simulink subsystem "Final_Project_PreBusUnpack_20260601_105527"  (R2024a)
settings: Solver=VariableStepAuto  StartTime=0.0  StopTime=10.0  RelTol=1e-3
values from neighbouring files (symbols this model uses):
  D = hypot(Ep(:,1)-Tp(:,1)',Ep(:,2)-Tp(:,2)')    [pp_compare_stage.m]    (also in pp_diag_path.m; pp_t09_clear.m = hypot(Ep(:,1)-Tperim(:,1)', Ep(:,2)-Tperim(:,2)'); pp_tune2.m)
undefined symbols (not defined in the file or in its folder): waypoints
libraries: CarMaker4SL x116, simulink x1
(part 4 of 7)

== matlab function Final_Project_PreBusUnpack_20260601_105527/Driving_Module_Ver.3_PSH/Subsystem/Ego_Detector ==
  data: ego_state input; ego_lane_id output; lanes input; target_lane_fb input; ego_cross_track_err output; ego_head_err output; ego_max_curvature output; park_cmd input
function [ego_lane_id, ego_cross_track_err, ego_head_err, ego_max_curvature] = Ego_Detector(ego_state, lanes, target_lane_fb, park_cmd)
%#codegen

    % ============================================================
    % 1. EgoStateBus unpack
    % ============================================================
    ego_x   = ego_state.Car_Fr1_tx;
    ego_y   = ego_state.Car_Fr1_ty;
    ego_yaw = ego_state.Car_Fr1_rz;

    % ============================================================
    % 2. ParsedLaneBus unpack - 5차선
    % ============================================================
    x1 = lanes.x1;  y1 = lanes.y1;
    x2 = lanes.x2;  y2 = lanes.y2;
    x3 = lanes.x3;  y3 = lanes.y3;
    x4 = lanes.x4;  y4 = lanes.y4;
    x5 = lanes.x5;  y5 = lanes.y5;

    % lane5 좌측 보정
    L5_OFFSET = 1.0;
    x5 = x5 + L5_OFFSET;

    % ============================================================
    % 3. 현재 ego가 가장 가까운 차선 판단
    % ============================================================
    d1 = nearest_d2(x1, y1, ego_x, ego_y);
    d2 = nearest_d2(x2, y2, ego_x, ego_y);
    d3 = nearest_d2(x3, y3, ego_x, ego_y);
    d4 = nearest_d2(x4, y4, ego_x, ego_y);
    d5 = nearest_d2(x5, y5, ego_x, ego_y);

    ego_lane_id = int32(1);
    dmin = d1;

    if d2 < dmin
        dmin = d2;
        ego_lane_id = int32(2);
    end

    if d3 < dmin
        dmin = d3;
        ego_lane_id = int32(3);
    end

    if d4 < dmin
        dmin = d4;
        ego_lane_id = int32(4);
    end

    if d5 < dmin
        ego_lane_id = int32(5);
    end

    % ============================================================
    % 4. target_lane 보호
    % ============================================================
    target_lane = int32(target_lane_fb);

    if target_lane < int32(1)
        target_lane = int32(1);
    elseif target_lane > int32(5)
        target_lane = int32(5);
    end

    % ============================================================
    % 5. 주차 진입 구간에서는 preview step 축소
    % ============================================================
    if park_cmd == int32(1) && ...
       (target_lane == int32(4) || target_lane == int32(5))
        LOOK_STEP = int32(2);
    else
        LOOK_STEP = int32(5);
    end

    % ============================================================
    % 6. target lane 기준 오차 / 곡률 계산
    % ============================================================
    if target_lane == int32(1)

        [ego_cross_track_err, ego_head_err, ego_max_curvature] = process_lane_closed( ...
            x1, y1, ego_x, ego_y, ego_yaw, LOOK_STEP);

    elseif target_lane == int32(2)

        [ego_cross_track_err, ego_head_err, ego_max_curvature] = process_lane_closed( ...
            x2, y2, ego_x, ego_y, ego_yaw, LOOK_STEP);

    elseif target_lane == int32(3)

        [ego_cross_track_err, ego_head_err, ego_max_curvature] = process_lane_closed( ...
            x3, y3, ego_x, ego_y, ego_yaw, LOOK_STEP);

    elseif target_lane == int32(4)

        [ego_cross_track_err, ego_head_err, ego_max_curvature] = process_lane_open( ...
            x4, y4, ego_x, ego_y, ego_yaw, LOOK_STEP);

    else

        [ego_cross_track_err, ego_head_err, ego_max_curvature] = process_lane_open( ...
            x5, y5, ego_x, ego_y, ego_yaw, LOOK_STEP);

    end

end


function d2 = nearest_d2(xa, ya, ex, ey)
%#codegen

    d2 = 1e12;
    N  = int32(numel(xa));

    for i = 1:N
        dxk = xa(i) - ex;
        dyk = ya(i) - ey;
        v   = dxk*dxk + dyk*dyk;

        if v < d2
            d2 = v;
        end
    end

end


function [ego_cross_track_err, ego_head_err, ego_max_curvature] = process_lane_open(xa, ya, ex, ey, eyaw, LOOK_STEP)
%#codegen

    N = int32(numel(xa));

    best_i  = int32(1);
    best_d2 = 1e12;

    for i = 1:N
        dxk = xa(i) - ex;
        dyk = ya(i) - ey;
        v   = dxk*dxk + dyk*dyk;

        if v < best_d2
            best_d2 = v;
            best_i  = i;
        end
    end

    look_i = best_i + LOOK_STEP;

    if look_i > N
        look_i = N;
    end

    if look_i > best_i

        path_yaw = atan2( ...
            ya(look_i) - ya(best_i), ...
            xa(look_i) - xa(best_i));

    elseif best_i > int32(1)

        path_yaw = atan2( ...
            ya(best_i) - ya(best_i - int32(1)), ...
            xa(best_i) - xa(best_i - int32(1)));

    else

        path_yaw = eyaw;

    end

    dxr = ex - xa(best_i);
    dyr = ey - ya(best_i);

    ego_cross_track_err = -sin(path_yaw) * dxr + cos(path_yaw) * dyr;

    ego_head_err = wrap_pi(path_yaw - eyaw);

    ego_max_curvature = 0.0;
    STEP = int32(5);

    for kk = 0:4
        base_i = best_i + int32(kk) * STEP;

        i1 = base_i;
        i2 = base_i + STEP;
        i3 = base_i + int32(2) * STEP;

        if i1 > N
            i1 = N;
        end

        if i2 > N
            i2 = N;
        end

        if i3 > N
            i3 = N;
        end

        if i1 < i2 && i2 < i3

            yaw1 = atan2( ...
                ya(i2) - ya(i1), ...
                xa(i2) - xa(i1));

            yaw2 = atan2( ...
                ya(i3) - ya(i2), ...
                xa(i3) - xa(i2));

            dyaw = wrap_pi(yaw2 - yaw1);

            ds = sqrt( ...
                (xa(i3) - xa(i1))^2 + ...
                (ya(i3) - ya(i1))^2);

            if ds > 0.1
                kappa = abs(dyaw) / ds;

                if kappa > ego_max_curvature
                    ego_max_curvature = kappa;
                end
            end
        end
    end

end


function [ego_cross_track_err, ego_head_err, ego_max_curvature] = process_lane_closed(xa, ya, ex, ey, eyaw, LOOK_STEP)
%#codegen

    N = int32(numel(xa));

    best_i  = int32(1);
    best_d2 = 1e12;

    for i = 1:N
        dxk = xa(i) - ex;
        dyk = ya(i) - ey;
        v   = dxk*dxk + dyk*dyk;

        if v < best_d2
            best_d2 = v;
            best_i  = i;
        end
    end

    look_i = wrap_idx(best_i + LOOK_STEP, N);

    path_yaw = atan2( ...
        ya(look_i) - ya(best_i), ...
        xa(look_i) - xa(best_i));

    dxr = ex - xa(best_i);
    dyr = ey - ya(best_i);

    ego_cross_track_err = -sin(path_yaw) * dxr + cos(path_yaw) * dyr;

    ego_head_err = wrap_pi(path_yaw - eyaw);

    ego_max_curvature = 0.0;
    STEP = int32(5);

    for kk = 0:4
        base_i = wrap_idx(best_i + int32(kk) * STEP, N);

        i1 = base_i;
        i2 = wrap_idx(base_i + STEP, N);
        i3 = wrap_idx(base_i + int32(2) * STEP, N);

        yaw1 = atan2( ...
            ya(i2) - ya(i1), ...
            xa(i2) - xa(i1));

        yaw2 = atan2( ...
            ya(i3) - ya(i2), ...
            xa(i3) - xa(i2));

        dyaw = wrap_pi(yaw2 - yaw1);

        ds = sqrt( ...
            (xa(i3) - xa(i1))^2 + ...
            (ya(i3) - ya(i1))^2);

        if ds > 0.1
            kappa = abs(dyaw) / ds;

            if kappa > ego_max_curvature
                ego_max_curvature = kappa;
            end
        end
    end

end


function idx = wrap_idx(idx_in, N)
%#codegen
    idx = idx_in;

    while idx > N
        idx = idx - N;
    end

    while idx < int32(1)
        idx = idx + N;
    end

end


function a = wrap_pi(a)
%#codegen

    while a > pi
        a = a - 2.0*pi;
    end

    while a < -pi
        a = a + 2.0*pi;
    end

end

== stateflow chart Final_Project_PreBusUnpack_20260601_105527/Chart ==
  (default) -> (junction 1)
  (junction 1) -> (junction 3) [order 1] : [mod(i,10) == 0]
      | {do_Logic_10ms;}
  (junction 1) -> (junction 7) [order 2]
  (junction 3) -> (junction 5)
  (junction 5) -> (junction 7)
  (junction 7) -> (junction 10)
  (junction 10) -> (junction 12) [order 1] : [mod(i, 50) == 0]
      | {do_Logic_50ms;}
  (junction 10) -> (junction 18) [order 2]
  (junction 12) -> (junction 16)
  (junction 16) -> (junction 18)
  (junction 18) -> (junction 25)
  (junction 25) -> (junction 27) [order 1] : [mod(i,100) == 0]
      | {do_Logic_100ms;}
  (junction 25) -> (junction 21) [order 2]
  (junction 27) -> (junction 29) : {i = 0;}
  (junction 29) -> (junction 21)
  (junction 21) -> (junction 32) : {i = i +1;}
  data: i local =0
  events: do_Logic_10ms output FUNCTION_CALL_EVENT; do_Logic_50ms output FUNCTION_CALL_EVENT; do_Logic_100ms output FUNCTION_CALL_EVENT

== matlab function Final_Project_PreBusUnpack_20260601_105527/Driving_Module_Ver.3_PSH/Subsystem/Traffic_Detector ==
  data: ego_state input Bus: EgoStateBus; lead_dist output double; lanes input Bus: ParsedLaneBus; traffic input; target_speed input double; ego_lane_id input int32; lead_speed output double; left_clear output boolean; right_clear output boolean
function [lead_dist, lead_speed, left_clear, right_clear] = Traffic_Detector(ego_state, lanes, traffic, target_speed, ego_lane_id)
%#codegen
% traffic : Obstacle_Info_Bus
% 내부 구조 예:
%   traffic.t16.x, traffic.t16.y, traffic.t16.vx, traffic.t16.vy
%   ...
%   traffic.t28.x, traffic.t28.y, traffic.t28.vx, traffic.t28.vy
%
% 주의:
%   target_speed는 배선 호환용으로 남겨두지만, 거리 판단에는 ego_v를 사용함.

    unused_target_speed = target_speed; %#ok<NASGU>

    % ============================================================
    % 0. 출력 초기화
    % ============================================================
    lead_dist   = 1e9;
    lead_speed  = 0.0;
    left_clear  = true;
    right_clear = true;
    ego_lane    = int32(ego_lane_id);

    % ============================================================
    % 1. Ego unpack
    % ============================================================
    ego_x = ego_state.Car_Fr1_tx;
    ego_y = ego_state.Car_Fr1_ty;
    ego_v = ego_state.Ego_V;

    % ============================================================
    % 2. Lane unpack - 5차선
    % ============================================================
    x1 = lanes.x1; y1 = lanes.y1;
    x2 = lanes.x2; y2 = lanes.y2;
    x3 = lanes.x3; y3 = lanes.y3;
    x4 = lanes.x4; y4 = lanes.y4;
    x5 = lanes.x5; y5 = lanes.y5;

    % detector와 lane5 기준을 맞추기 위한 보정
    L5_OFFSET = 1.0;
    x5 = x5 + L5_OFFSET;

    % ============================================================
    % 3. Ego 속도 기반 가변 탐색/안전거리
    % ============================================================
    v_ego_gap = abs(ego_v);

    if v_ego_gap > 60.0
        v_ego_gap = v_ego_gap / 3.6;
    end

    LOOK_FRONT = calcLookFront(v_ego_gap);

    CLEAR_BACK_MIN = 5.0;
    CLEAR_BACK_TG  = 0.5;
    CLEAR_BACK_MAX = 35.0;

    CLEAR_BACK = CLEAR_BACK_MIN + CLEAR_BACK_TG * v_ego_gap;

    if CLEAR_BACK > CLEAR_BACK_MAX
        CLEAR_BACK = CLEAR_BACK_MAX;
    end

    CLEAR_FRONT_MIN = 15.0;
    CLEAR_FRONT_TG  = 0.9;
    CLEAR_FRONT_MAX = 70.0;

    CLEAR_FRONT = CLEAR_FRONT_MIN + CLEAR_FRONT_TG * v_ego_gap;

    if CLEAR_FRONT > CLEAR_FRONT_MAX
        CLEAR_FRONT = CLEAR_FRONT_MAX;
    end

    % ============================================================
    % 4. Init
    % ============================================================
    lead_dist  = 1e9;
    lead_speed = v_ego_gap;

    left_clear  = true;
    right_clear = true;

    if ego_lane >= int32(5)
        left_clear = false;
    end

    if ego_lane <= int32(1)
        right_clear = false;
    end

    % ============================================================
    % 5. Traffic_Info_16_Bus ~ Traffic_Info_28_Bus 직접 처리
    % ============================================================
    [lead_dist, lead_speed, left_clear, right_clear] = check_one_signal( ...
        traffic.t16.x, traffic.t16.y, traffic.t16.vx, traffic.t16.vy, true, ...
        ego_x, ego_y, ego_lane, ...
        x1,y1,x2,y2,x3,y3,x4,y4,x5,y5, ...
        lead_dist, lead_speed, left_clear, right_clear, ...
        LOOK_FRONT, CLEAR_BACK, CLEAR_FRONT);

    [lead_dist, lead_speed, left_clear, right_clear] = check_one_signal( ...
        traffic.t17.x, traffic.t17.y, traffic.t17.vx, traffic.t17.vy, true, ...
        ego_x, ego_y, ego_lane, ...
        x1,y1,x2,y2,x3,y3,x4,y4,x5,y5, ...
        lead_dist, lead_speed, left_clear, right_clear, ...
        LOOK_FRONT, CLEAR_BACK, CLEAR_FRONT);

    [lead_dist, lead_speed, left_clear, right_clear] = check_one_signal( ...
        traffic.t18.x, traffic.t18.y, traffic.t18.vx, traffic.t18.vy, true, ...
        ego_x, ego_y, ego_lane, ...
        x1,y1,x2,y2,x3,y3,x4,y4,x5,y5, ...
        lead_dist, lead_speed, left_clear, right_clear, ...
        LOOK_FRONT, CLEAR_BACK, CLEAR_FRONT);

    [lead_dist, lead_speed, left_clear, right_clear] = check_one_signal( ...
        traffic.t19.x, traffic.t19.y, traffic.t19.vx, traffic.t19.vy, true, ...
        ego_x, ego_y, ego_lane, ...
        x1,y1,x2,y2,x3,y3,x4,y4,x5,y5, ...
        lead_dist, lead_speed, left_clear, right_clear, ...
        LOOK_FRONT, CLEAR_BACK, CLEAR_FRONT);

    [lead_dist, lead_speed, left_clear, right_clear] = check_one_signal( ...
        traffic.t20.x, traffic.t20.y, traffic.t20.vx, traffic.t20.vy, true, ...
        ego_x, ego_y, ego_lane, ...
        x1,y1,x2,y2,x3,y3,x4,y4,x5,y5, ...
        lead_dist, lead_speed, left_clear, right_clear, ...
        LOOK_FRONT, CLEAR_BACK, CLEAR_FRONT);

    [lead_dist, lead_speed, left_clear, right_clear] = check_one_signal( ...
        traffic.t21.x, traffic.t21.y, traffic.t21.vx, traffic.t21.vy, true, ...
        ego_x, ego_y, ego_lane, ...
        x1,y1,x2,y2,x3,y3,x4,y4,x5,y5, ...
        lead_dist, lead_speed, left_clear, right_clear, ...
        LOOK_FRONT, CLEAR_BACK, CLEAR_FRONT);

    [lead_dist, lead_speed, left_clear, right_clear] = check_one_signal( ...
        traffic.t22.x, traffic.t22.y, traffic.t22.vx, traffic.t22.vy, true, ...
        ego_x, ego_y, ego_lane, ...
        x1,y1,x2,y2,x3,y3,x4,y4,x5,y5, ...
        lead_dist, lead_speed, left_clear, right_clear, ...
        LOOK_FRONT, CLEAR_BACK, CLEAR_FRONT);

    [lead_dist, lead_speed, left_clear, right_clear] = check_one_signal( ...
        traffic.t23.x, traffic.t23.y, traffic.t23.vx, traffic.t23.vy, true, ...
        ego_x, ego_y, ego_lane, ...
        x1,y1,x2,y2,x3,y3,x4,y4,x5,y5, ...
        lead_dist, lead_speed, left_clear, right_clear, ...
        LOOK_FRONT, CLEAR_BACK, CLEAR_FRONT);

    [lead_dist, lead_speed, left_clear, right_clear] = check_one_signal( ...
        traffic.t24.x, traffic.t24.y, traffic.t24.vx, traffic.t24.vy, true, ...
        ego_x, ego_y, ego_lane, ...
        x1,y1,x2,y2,x3,y3,x4,y4,x5,y5, ...
        lead_dist, lead_speed, left_clear, right_clear, ...
        LOOK_FRONT, CLEAR_BACK, CLEAR_FRONT);

    [lead_dist, lead_speed, left_clear, right_clear] = check_one_signal( ...
        traffic.t25.x, traffic.t25.y, traffic.t25.vx, traffic.t25.vy, true, ...
        ego_x, ego_y, ego_lane, ...
        x1,y1,x2,y2,x3,y3,x4,y4,x5,y5, ...
        lead_dist, lead_speed, left_clear, right_clear, ...
        LOOK_FRONT, CLEAR_BACK, CLEAR_FRONT);

    [lead_dist, lead_speed, left_clear, right_clear] = check_one_signal( ...
        traffic.t26.x, traffic.t26.y, traffic.t26.vx, traffic.t26.vy, true, ...
        ego_x, ego_y, ego_lane, ...
        x1,y1,x2,y2,x3,y3,x4,y4,x5,y5, ...
        lead_dist, lead_speed, left_clear, right_clear, ...
        LOOK_FRONT, CLEAR_BACK, CLEAR_FRONT);

    [lead_dist, lead_speed, left_clear, right_clear] = check_one_signal( ...
        traffic.t27.x, traffic.t27.y, traffic.t27.vx, traffic.t27.vy, true, ...
        ego_x, ego_y, ego_lane, ...
        x1,y1,x2,y2,x3,y3,x4,y4,x5,y5, ...
        lead_dist, lead_speed, left_clear, right_clear, ...
        LOOK_FRONT, CLEAR_BACK, CLEAR_FRONT);

    [lead_dist, lead_speed, left_clear, right_clear] = check_one_signal( ...
        traffic.t28.x, traffic.t28.y, traffic.t28.vx, traffic.t28.vy, true, ...
        ego_x, ego_y, ego_lane, ...
        x1,y1,x2,y2,x3,y3,x4,y4,x5,y5, ...
        lead_dist, lead_speed, left_clear, right_clear, ...
        LOOK_FRONT, CLEAR_BACK, CLEAR_FRONT);

end


function LOOK_FRONT = calcLookFront(v)
%#codegen
    v = abs(v);

    if v > 60.0
        v = v / 3.6;
    end

    V_HIGH = 80.0 / 3.6;

    if v < V_HIGH
        LOOK_FRONT = 25.0 + 1.0 * v;
    else
        LOOK_FRONT = 25.0 + 1.0 * V_HIGH + 10.0 * (v - V_HIGH);
    end

    if LOOK_FRONT > 120.0
        LOOK_FRONT = 120.0;
    end
end


function [lead_dist, lead_speed, left_clear, right_clear] = check_one_signal( ...
    obj_x, obj_y, obj_vx, obj_vy, valid, ...
    ego_x, ego_y, ego_lane_id, ...
    x1,y1,x2,y2,x3,y3,x4,y4,x5,y5, ...
    lead_dist, lead_speed, left_clear, right_clear, ...
    LOOK_FRONT, CLEAR_BACK, CLEAR_FRONT)
%#codegen

    if ~valid
        return;
    end

    [lead_dist, lead_speed, left_clear, right_clear] = check_one_vehicle( ...
        ego_x, ego_y, ego_lane_id, ...
        obj_x, obj_y, obj_vx, obj_vy, ...
        x1,y1,x2,y2,x3,y3,x4,y4,x5,y5, ...
        lead_dist, lead_speed, left_clear, right_clear, ...
        LOOK_FRONT, CLEAR_BACK, CLEAR_FRONT);

end


function [lead_dist, lead_speed, left_clear, right_clear] = check_one_vehicle( ...
    ego_x, ego_y, ego_lane_id, ...
    obj_x, obj_y, obj_vx, obj_vy, ...
    x1, y1, x2, y2, x3, y3, x4, y4, x5, y5, ...
    lead_dist, lead_speed, left_clear, right_clear, ...
    LOOK_FRONT, CLEAR_BACK, CLEAR_FRONT)
%#codegen

    [obj_lane_id, obj_idx] = nearest_lane_id( ...
        obj_x, obj_y, ...
        x1, y1, x2, y2, x3, y3, x4, y4, x5, y5);

    if obj_lane_id == ego_lane_id

        ego_idx = nearest_idx_by_lane( ...
            ego_lane_id, ego_x, ego_y, ...
            x1, y1, x2, y2, x3, y3, x4, y4, x5, y5);

        s_rel = arc_dist_forward_by_lane( ...
            ego_lane_id, ego_idx, obj_idx, ...
            x1, y1, x2, y2, x3, y3, x4, y4, x5, y5);

        if s_rel > 0.0 && s_rel < LOOK_FRONT
            if s_rel < lead_dist
                lead_dist  = s_rel;
                lead_speed = sqrt(obj_vx*obj_vx + obj_vy*obj_vy);
            end
        end
    end

    if obj_lane_id == ego_lane_id + int32(1)

        ego_idx_adj = nearest_idx_by_lane( ...
            obj_lane_id, ego_x, ego_y, ...
            x1, y1, x2, y2, x3, y3, x4, y4, x5, y5);

        is_close = is_close_on_adj_lane( ...
            obj_lane_id, ego_idx_adj, obj_idx, ...
            CLEAR_BACK, CLEAR_FRONT, ...
            x1, y1, x2, y2, x3, y3, x4, y4, x5, y5);

        if is_close
            left_clear = false;
        end

    elseif obj_lane_id == ego_lane_id - int32(1)

        ego_idx_adj = nearest_idx_by_lane( ...
            obj_lane_id, ego_x, ego_y, ...
            x1, y1, x2, y2, x3, y3, x4, y4, x5, y5);

        is_close = is_close_on_adj_lane( ...
            obj_lane_id, ego_idx_adj, obj_idx, ...
            CLEAR_BACK, CLEAR_FRONT, ...
            x1, y1, x2, y2, x3, y3, x4, y4, x5, y5);

        if is_close
            right_clear = false;
        end
    end

end


function [lane_id, best_idx] = nearest_lane_id(px, py, x1, y1, x2, y2, x3, y3, x4, y4, x5, y5)
%#codegen

    [idx1, d1] = nearest_idx_d2(x1, y1, px, py);
    [idx2, d2] = nearest_idx_d2(x2, y2, px, py);
    [idx3, d3] = nearest_idx_d2(x3, y3, px, py);
    [idx4, d4] = nearest_idx_d2(x4, y4, px, py);
    [idx5, d5] = nearest_idx_d2(x5, y5, px, py);

    lane_id  = int32(1);
    best_idx = idx1;
    best_d2  = d1;

    if d2 < best_d2
        lane_id  = int32(2);
        best_idx = idx2;
        best_d2  = d2;
    end

    if d3 < best_d2
        lane_id  = int32(3);
        best_idx = idx3;
        best_d2  = d3;
    end

    if d4 < best_d2
        lane_id  = int32(4);
        best_idx = idx4;
        best_d2  = d4;
    end

    if d5 < best_d2
        lane_id  = int32(5);
        best_idx = idx5;
    end

end


function idx = nearest_idx_by_lane(lane_id, px, py, x1, y1, x2, y2, x3, y3, x4, y4, x5, y5)
%#codegen

    if lane_id == int32(1)
        [idx, ~] = nearest_idx_d2(x1, y1, px, py);
    elseif lane_id == int32(2)
        [idx, ~] = nearest_idx_d2(x2, y2, px, py);
    elseif lane_id == int32(3)
        [idx, ~] = nearest_idx_d2(x3, y3, px, py);
    elseif lane_id == int32(4)
        [idx, ~] = nearest_idx_d2(x4, y4, px, py);
    else
        [idx, ~] = nearest_idx_d2(x5, y5, px, py);
    end

end


function [best_i, best_d2] = nearest_idx_d2(xa, ya, px, py)
%#codegen

    best_i  = int32(1);
    best_d2 = 1e12;
    N = int32(numel(xa));

    for i = 1:N
        dx = xa(i) - px;
        dy = ya(i) - py;
        d2 = dx*dx + dy*dy;

        if d2 < best_d2
            best_d2 = d2;
            best_i  = i;
        end
    end

end


function ds = arc_dist_forward_by_lane(lane_id, idx_from, idx_to, ...
    x1, y1, x2, y2, x3, y3, x4, y4, x5, y5)
%#codegen

    if lane_id == int32(1)
        ds = arc_dist_forward_closed(x1, y1, idx_from, idx_to);
    elseif lane_id == int32(2)
        ds = arc_dist_forward_closed(x2, y2, idx_from, idx_to);
    elseif lane_id == int32(3)
        ds = arc_dist_forward_closed(x3, y3, idx_from, idx_to);
    elseif lane_id == int32(4)
        ds = arc_dist_open(x4, y4, idx_from, idx_to);
    else
        ds = arc_dist_open(x5, y5, idx_from, idx_to);
    end

end


function ds = arc_dist_forward_closed(xa, ya, idx_from, idx_to)
%#codegen

    ds = 0.0;
    N = int32(numel(xa));

    if idx_to == idx_from
        ds = 0.0;
        return;
    end

    if idx_to > idx_from

        for i = idx_from:(idx_to - int32(1))
            dx = xa(i+1) - xa(i);
            dy = ya(i+1) - ya(i);
            ds = ds + sqrt(dx*dx + dy*dy);
        end

    else

        for i = idx_from:(N - int32(1))
            dx = xa(i+1) - xa(i);
            dy = ya(i+1) - ya(i);
            ds = ds + sqrt(dx*dx + dy*dy);
        end

        dx = xa(1) - xa(N);
        dy = ya(1) - ya(N);
        ds = ds + sqrt(dx*dx + dy*dy);

        for i = int32(1):(idx_to - int32(1))
            dx = xa(i+1) - xa(i);
            dy = ya(i+1) - ya(i);
            ds = ds + sqrt(dx*dx + dy*dy);
        end

    end

end


function is_close = is_close_on_adj_lane(lane_id, idx_from, idx_to, ...
    CLEAR_BACK, CLEAR_FRONT, ...
    x1, y1, x2, y2, x3, y3, x4, y4, x5, y5)
%#codegen

    is_close = false;

    if lane_id == int32(1)

        fwd_dist  = arc_dist_forward_closed(x1, y1, idx_from, idx_to);
        total_len = arc_length_closed(x1, y1);
        back_dist = total_len - fwd_dist;

        if fwd_dist < CLEAR_FRONT || back_dist < CLEAR_BACK
            is_close = true;
        end

    elseif lane_id == int32(2)

        fwd_dist  = arc_dist_forward_closed(x2, y2, idx_from, idx_to);
        total_len = arc_length_closed(x2, y2);
        back_dist = total_len - fwd_dist;

        if fwd_dist < CLEAR_FRONT || back_dist < CLEAR_BACK
            is_close = true;
        end

    elseif lane_id == int32(3)

        fwd_dist  = arc_dist_forward_closed(x3, y3, idx_from, idx_to);
        total_len = arc_length_closed(x3, y3);
        back_dist = total_len - fwd_dist;

        if fwd_dist < CLEAR_FRONT || back_dist < CLEAR_BACK
            is_close = true;
        end

    elseif lane_id == int32(4)

        s_rel = arc_dist_open(x4, y4, idx_from, idx_to);

        if s_rel > -CLEAR_BACK && s_rel < CLEAR_FRONT
            is_close = true;
        end

    else

        s_rel = arc_dist_open(x5, y5, idx_from, idx_to);

        if s_rel > -CLEAR_BACK && s_rel < CLEAR_FRONT
            is_close = true;
        end

    end

end


function total_len = arc_length_closed(xa, ya)
%#codegen

    total_len = 0.0;
    N = int32(numel(xa));

    for i = int32(1):(N - int32(1))
        dx = xa(i+1) - xa(i);
        dy = ya(i+1) - ya(i);
        total_len = total_len + sqrt(dx*dx + dy*dy);
    end

    dx = xa(1) - xa(N);
    dy = ya(1) - ya(N);
    total_len = total_len + sqrt(dx*dx + dy*dy);

end


function ds = arc_dist_open(xa, ya, idx_from, idx_to)
%#codegen

    ds = 0.0;

    if idx_to == idx_from

        ds = 0.0;

    elseif idx_to > idx_from

        for i = idx_from:(idx_to - int32(1))
            dx = xa(i+1) - xa(i);
            dy = ya(i+1) - ya(i);
            ds = ds + sqrt(dx*dx + dy*dy);
        end

    else

        for i = idx_to:(idx_from - int32(1))
            dx = xa(i+1) - xa(i);
            dy = ya(i+1) - ya(i);
            ds = ds - sqrt(dx*dx + dy*dy);
        end

    end

end

== matlab function Final_Project_PreBusUnpack_20260601_105527/Driving_Module_Ver.3_PSH/Subsystem/Decision ==
  data: ego_cross_track_err input; lead_dist input; left_clear input; right_clear input; submission_state input; desired_lane output int32; ego_state input; drive_state output; lane_settled output; ego_lane_id input
function [desired_lane, drive_state, lane_settled] = Decision(ego_cross_track_err, lead_dist, left_clear, right_clear, submission_state, ego_state, ego_lane_id)
%#codegen

    % ============================================================
    % Parameters
    % ============================================================
    LCHG_TRIG_D     = 25.0;
    LAT_ARRIVED     = 0.5;

    MIN_LANE        = int32(1);
    MAX_NORMAL_LANE = int32(3);
    MAX_LANE        = int32(5);

    MODE_ACC  = int32(0);
    MODE_LCHG = int32(1);
    MODE_PARK = int32(2);

    MIN_LCHG_STEP = int32(120);

    PARK_FRONT_HOLD_D = 8.0;

    % ============================================================
    % Ego position
    % ============================================================
    ego_x = ego_state.Car_Fr1_tx;
    ego_y = ego_state.Car_Fr1_ty;

    % ============================================================
    % Parking entry waypoints
    % ============================================================
    L4_X = -46.856;  L4_Y = 15.842;
    L5_X =  -6.845;  L5_Y = 12.658;

    DIST_PREP_L3  = 150.0;
    DIST_ENTER_L4 = 20.0;
    DIST_ENTER_L5 =  8.0;

    % ============================================================
    % Persistent states
    % ============================================================
    persistent target_lane_p mode_p lchg_timer_p park_state did_init

    if isempty(did_init)
        target_lane_p = int32(2);
        mode_p        = MODE_ACC;
        lchg_timer_p  = int32(0);
        park_state    = int32(0);
        did_init      = true;
    end

    % ============================================================
    % 기본 출력
    % lane_settled은 차선변경 완료 순간에만 true pulse
    % ============================================================
    desired_lane  = target_lane_p;
    drive_state   = mode_p;
    lane_settled  = false;

    % ============================================================
    % Safety clamp
    % ============================================================
    if target_lane_p < MIN_LANE
        target_lane_p = MIN_LANE;
    elseif target_lane_p > MAX_LANE
        target_lane_p = MAX_LANE;
    end

    % ============================================================
    % Distance to parking waypoints
    % ============================================================
    dist_l4 = sqrt((ego_x - L4_X)^2 + (ego_y - L4_Y)^2);
    dist_l5 = sqrt((ego_x - L5_X)^2 + (ego_y - L5_Y)^2);

    % ============================================================
    % Parking command latch
    %
    % 톨게이트 selector가 target_lane을 1차선으로 override했기 때문에
    % decision 내부 target_lane_p와 실제 차량 차선이 다를 수 있음.
    % submission_state가 처음 들어오는 순간 target_lane_p를 ego_lane_id로 동기화.
    % ============================================================
    if park_state == int32(0)
        if submission_state == int32(1)

            target_lane_p = int32(ego_lane_id);

            if target_lane_p < int32(1)
                target_lane_p = int32(1);
            elseif target_lane_p > int32(3)
                target_lane_p = int32(3);
            end

            mode_p       = MODE_ACC;
            lchg_timer_p = int32(0);

            park_state = int32(1);
        end
    end

    % ============================================================
    % 주차장 진입 중 새 차선변경 시작 가능 여부
    % ============================================================
    front_ok_for_new_lchg = true;

    if lead_dist < PARK_FRONT_HOLD_D
        front_ok_for_new_lchg = false;
    end

    % ============================================================
    % Parking state machine
    % ============================================================
    if park_state == int32(1)

        if mode_p ~= MODE_LCHG && ...
           dist_l4 < DIST_PREP_L3 && ...
           target_lane_p ~= int32(3) && ...
           front_ok_for_new_lchg

            next_lane = target_lane_p;

            if target_lane_p < int32(3)
                next_lane = target_lane_p + int32(1);
            elseif target_lane_p > int32(3)
                next_lane = target_lane_p - int32(1);
            end

            if can_change_one_lane(target_lane_p, next_lane, left_clear, right_clear)

                target_lane_p = next_lane;
                mode_p        = MODE_LCHG;
                lchg_timer_p  = MIN_LCHG_STEP;

            end
        end

        if mode_p ~= MODE_LCHG && ...
           dist_l4 < DIST_ENTER_L4 && ...
           target_lane_p == int32(3) && ...
           front_ok_for_new_lchg

            next_lane = int32(4);

            if can_change_one_lane(target_lane_p, next_lane, left_clear, right_clear)

                target_lane_p = next_lane;
                mode_p        = MODE_LCHG;
                lchg_timer_p  = MIN_LCHG_STEP;
                park_state    = int32(2);

            end
        end

    elseif park_state == int32(2)

        if target_lane_p == int32(4) && mode_p ~= MODE_LCHG
            park_state = int32(3);
        end

    elseif park_state == int32(3)

        if mode_p ~= MODE_LCHG && ...
           dist_l5 < DIST_ENTER_L5 && ...
           front_ok_for_new_lchg

            next_lane = int32(5);

            if can_change_one_lane(target_lane_p, next_lane, left_clear, right_clear)

                target_lane_p = next_lane;
                mode_p        = MODE_LCHG;
                lchg_timer_p  = MIN_LCHG_STEP;
                park_state    = int32(4);

            end
        end

    elseif park_state == int32(4)

        if target_lane_p == int32(5) && mode_p ~= MODE_LCHG
            mode_p     = MODE_PARK;
            park_state = int32(5);
        end

    elseif park_state >= int32(5)

        mode_p = MODE_PARK;
    end

    % ============================================================
    % Parking 진행 중이면 일반 주행 로직을 타지 않음
    % ============================================================
    if park_state > int32(0)

        if mode_p == MODE_LCHG

            if lchg_timer_p > int32(0)

                lchg_timer_p = lchg_timer_p - int32(1);

            else

                if abs(ego_cross_track_err) < LAT_ARRIVED
                    mode_p       = MODE_ACC;
                    lane_settled = true;
                end

            end
        end

        desired_lane = target_lane_p;
        drive_state  = mode_p;
        return;
    end

    % ============================================================
    % 일반 주행 로직
    % ============================================================
    if mode_p == MODE_ACC

        if lead_dist < LCHG_TRIG_D

            if left_clear && target_lane_p < MAX_NORMAL_LANE

                target_lane_p = target_lane_p + int32(1);
                mode_p        = MODE_LCHG;
                lchg_timer_p  = MIN_LCHG_STEP;

            elseif right_clear && target_lane_p > MIN_LANE

                target_lane_p = target_lane_p - int32(1);
                mode_p        = MODE_LCHG;
                lchg_timer_p  = MIN_LCHG_STEP;

            end
        end

    else

        if lchg_timer_p > int32(0)

            lchg_timer_p = lchg_timer_p - int32(1);

        else

            if abs(ego_cross_track_err) < LAT_ARRIVED

                mode_p       = MODE_ACC;
                lane_settled = true;

            end
        end
    end

    % ============================================================
    % 갱신된 출력
    % ============================================================
    desired_lane = target_lane_p;
    drive_state  = mode_p;

end


function ok = can_change_one_lane(cur_lane, next_lane, left_clear, right_clear)
%#codegen

    ok = false;

    if next_lane == cur_lane

        ok = true;

    elseif next_lane == cur_lane + int32(1)

        if left_clear
            ok = true;
        end

    elseif next_lane == cur_lane - int32(1)

        if right_clear
            ok = true;
        end

    else

        ok = false;

    end

end

== matlab function Final_Project_PreBusUnpack_20260601_105527/Driving_Module_Ver.3_PSH/Subsystem/Tollgate_Selector ==
  data: ego_state input; target_lane_out output; tollgate_cmd input; desired_lane input; ego_lane_id input; ego_cross_track_err input; ego_max_curvature input; left_clear input; right_clear input; toll_speed_limit output; toll_target_lane_cmd input; toll_pass_speed_cmd input
function [target_lane_out, toll_speed_limit] = tollgate_selector( ...
    ego_state, tollgate_cmd, desired_lane, ego_lane_id, ego_cross_track_err, ego_max_curvature, left_clear, right_clear, ...
    toll_target_lane_cmd, toll_pass_speed_cmd)
%#codegen

    % ============================================================
    % Cmd 정의
    % 0 : Default
    % 1 : Parking
    % 2 : Tollgate
    % ============================================================
    CMD_TOLLGATE = int32(2);

    % ============================================================
    % 지정 톨게이트 차선
    % 외부 입력으로 받음
    % ============================================================
    TOLL_TARGET_LANE = int32(toll_target_lane_cmd);

    % ============================================================
    % 톨게이트 좌표
    % ============================================================
    G1_X = -176.212;
    G1_Y = -86.9523;

    G2_X = -172.724;
    G2_Y = -86.2036;

    G3_X = -169.207;
    G3_Y = -87.124;

    % ============================================================
    % 거리 / 속도 파라미터
    % ============================================================
    TOLL_REACHED_DIST = 6.0;
    SPEED_NONE        = 1.0e9;

    TOLL_APPROACH_SPEED = 50.0 / 3.6;
    TOLL_GAP_SPEED      = 30.0 / 3.6;
    TOLL_CRAWL_SPEED    = 5.0  / 3.6;
    TOLL_PASS_SPEED     = toll_pass_speed_cmd;

    % toll_pass_speed_cmd가 km/h로 들어오는 경우 보호
    if TOLL_PASS_SPEED > 20.0
        TOLL_PASS_SPEED = TOLL_PASS_SPEED / 3.6;
    end

    TOLL_APPROACH_DIST  = 100.0;

    LANE_CHANGE_DIST = 45.0;
    DIST_MARGIN      = 20.0;

    % ============================================================
    % 한 차선 이동 후 안정 판단
    % ============================================================
    LAT_SETTLE    = 0.6;
    MIN_HOLD_STEP = int32(80);    % 0.01초 기준 0.8초

    % ============================================================
    % 톨게이트 모드 진입 직후 대기
    % ============================================================
    ENTER_WAIT_STEP = int32(30);  % 0.01초 기준 0.3초 대기

    % ============================================================
    % 고속/커브 상황에서 차선변경 시작 억제
    % ============================================================
    LCHG_START_MAX_V = 55.0 / 3.6;
    CURVE_START_MAX  = 0.018;
    LOW_SPEED_ALLOW  = 35.0 / 3.6;

    % ============================================================
    % Ego unpack
    % ============================================================
    ego_x = ego_state.Car_Fr1_tx;
    ego_y = ego_state.Car_Fr1_ty;
    ego_v = ego_state.Ego_V;

    % ============================================================
    % persistent 상태
    % passed_p : 내부 톨게이트 통과 상태
    % ============================================================
    persistent passed_p prev_toll_p step_lane_p hold_count_p enter_wait_p did_init

    if isempty(did_init)
        passed_p     = false;
        prev_toll_p  = false;
        step_lane_p  = int32(2);
        hold_count_p = int32(0);
        enter_wait_p = int32(0);
        did_init     = true;
    end

    % ============================================================
    % 기본 출력
    % desired_lane은 parking 모드에서 4 또는 5가 될 수 있으므로
    % 여기서는 기본값을 절대 1~3으로 clamp하면 안 됨.
    % ============================================================
    target_lane_out  = int32(desired_lane);
    toll_speed_limit = SPEED_NONE;

    toll_now = (int32(tollgate_cmd) == CMD_TOLLGATE);

    % ============================================================
    % tollgate_cmd가 2로 처음 들어오는 순간 초기화
    % ============================================================
    if toll_now && ~prev_toll_p
        passed_p = false;

        % 진입 순간에는 기존 desired_lane을 유지
        step_lane_p  = clamp_toll_lane(desired_lane);
        hold_count_p = int32(0);
        enter_wait_p = ENTER_WAIT_STEP;
    end

    prev_toll_p = toll_now;

    % ============================================================
    % tollgate_cmd가 2가 아니면 톨게이트 개입 없음
    % ============================================================
    if ~toll_now
        passed_p         = false;
        toll_speed_limit = SPEED_NONE;

        hold_count_p     = int32(0);
        enter_wait_p     = int32(0);
        target_lane_out  = int32(desired_lane);
        return;
    end

    % ============================================================
    % 이미 톨게이트 통과 후인 경우
    % ============================================================
    if passed_p
        target_lane_out  = TOLL_TARGET_LANE;
        toll_speed_limit = SPEED_NONE;
        return;
    end

    % ============================================================
    % 선택된 톨게이트 좌표
    % ============================================================
    if TOLL_TARGET_LANE == int32(1)
        gate_x = G1_X;
        gate_y = G1_Y;
    elseif TOLL_TARGET_LANE == int32(2)
        gate_x = G2_X;
        gate_y = G2_Y;
    else
        gate_x = G3_X;
        gate_y = G3_Y;
    end

    % ============================================================
    % 톨게이트까지 거리
    % ============================================================
    dx = ego_x - gate_x;
    dy = ego_y - gate_y;
    dist_to_toll = sqrt(dx * dx + dy * dy);

    % ============================================================
    % 현재 차선 / 중간 목표 차선 정리
    % ============================================================
    current_lane = clamp_toll_lane(ego_lane_id);
    step_lane_p  = clamp_toll_lane(step_lane_p);

    % ============================================================
    % 속도 단위 방어
    % ============================================================
    v = ego_v;

    if v > 60.0
        v = v / 3.6;
    end

    % ============================================================
    % 고속/커브 차선변경 시작 조건
    % ============================================================
    speed_ok = (v <= LCHG_START_MAX_V);

    if ego_max_curvature <= CURVE_START_MAX
        curve_ok = true;
    elseif v <= LOW_SPEED_ALLOW
        curve_ok = true;
    else
        curve_ok = false;
    end

    start_lchg_ok = speed_ok && curve_ok;

    % ============================================================
    % 톨게이트 모드 진입 직후 보호 구간
    % ============================================================
    if enter_wait_p > int32(0)

        enter_wait_p = enter_wait_p - int32(1);

        target_lane_out  = int32(desired_lane);
        toll_speed_limit = SPEED_NONE;

        if ~speed_ok
            toll_speed_limit = TOLL_APPROACH_SPEED;
        end

        if ~curve_ok
            toll_speed_limit = TOLL_APPROACH_SPEED;
        end

        if dist_to_toll < TOLL_APPROACH_DIST
            if toll_speed_limit > TOLL_APPROACH_SPEED
                toll_speed_limit = TOLL_APPROACH_SPEED;
            end
        end

        if enter_wait_p == int32(0)
            step_lane_p  = current_lane;
            hold_count_p = int32(0);
        end

        return;
    end

    % ============================================================
    % 옆차선 clear 확인
    % ============================================================
    if step_lane_p > TOLL_TARGET_LANE
        side_clear_ok = (right_clear ~= 0);
    elseif step_lane_p < TOLL_TARGET_LANE
        side_clear_ok = (left_clear ~= 0);
    else
        side_clear_ok = true;
    end

    % ============================================================
    % Mandatory tollgate 속도 제한
    % ============================================================
    lanes_remaining = abs(double(current_lane) - double(TOLL_TARGET_LANE));

    if lanes_remaining > 0.0

        required_dist = lanes_remaining * LANE_CHANGE_DIST + DIST_MARGIN;

        toll_speed_limit = SPEED_NONE;

        if ~speed_ok
            toll_speed_limit = TOLL_APPROACH_SPEED;
        end

        if ~curve_ok
            toll_speed_limit = TOLL_APPROACH_SPEED;
        end

        if ~side_clear_ok
            toll_speed_limit = TOLL_GAP_SPEED;
        end

        if dist_to_toll < required_dist
            toll_speed_limit = TOLL_CRAWL_SPEED;
        end

    else

        if dist_to_toll < TOLL_APPROACH_DIST
            toll_speed_limit = TOLL_PASS_SPEED;
        else
            toll_speed_limit = SPEED_NONE;
        end
    end

    % ============================================================
    % 한 차선씩만 이동
    % ============================================================
    if step_lane_p ~= TOLL_TARGET_LANE

        if current_lane == step_lane_p

            if abs(ego_cross_track_err) < LAT_SETTLE
                hold_count_p = hold_count_p + int32(1);
            else
                hold_count_p = int32(0);
            end

            if hold_count_p >= MIN_HOLD_STEP && start_lchg_ok && side_clear_ok

                if step_lane_p < TOLL_TARGET_LANE
                    step_lane_p = step_lane_p + int32(1);
                elseif step_lane_p > TOLL_TARGET_LANE
                    step_lane_p = step_lane_p - int32(1);
                end

                step_lane_p  = clamp_toll_lane(step_lane_p);
                hold_count_p = int32(0);
            end

        else
            hold_count_p = int32(0);
        end
    end

    % ============================================================
    % 최종 출력 target_lane
    % ============================================================
    target_lane_out = step_lane_p;

    % ============================================================
    % 톨게이트 통과 판단
    % ============================================================
    if dist_to_toll < TOLL_REACHED_DIST
        passed_p = true;

        target_lane_out  = TOLL_TARGET_LANE;
        toll_speed_limit = SPEED_NONE;
    end

end


function lane = clamp_toll_lane(lane_in)
%#codegen
    lane = int32(lane_in);

    if lane < int32(1)
        lane = int32(1);
    elseif lane > int32(3)
        lane = int32(3);
    end
end
